simulink model "UAM_Status"  (R2024b)
settings: Solver=FixedStepAuto  StartTime=0.0  StopTime=10.0  RelTol=1e-3
libraries: simulink x1
settings Model: DataDictionary=UAM_data.sldd  Creator=admin  LastModifiedBy=admin
settings OptimizationCC: DefaultParameterBehavior=Inlined  EnhancedBackFolding=on  PassReuseOutputArgsAs=Individual arguments  ZeroExternalMemoryAtStartup=off  ZeroInternalMemoryAtStartup=off  OptimizeBlockOrder=speed  DifferentSizesBufferReuse=on  OptimizationCustomize=off  EfficientTunableParamExpr=on
settings DebuggingCC: ParameterTunabilityLossMsg=error
settings HardwareCC: ProdBitPerLong=64  ProdLargestAtomicInteger=LongLong  ProdLargestAtomicFloat=Double  ProdLongLongMode=on  ProdHWDeviceType=ARM Compatible->ARM Cortex-A (64-bit)
settings SFSimCC: MATLABDynamicMemAlloc=off
settings RTWCC: Description=Embedded Coder  SystemTargetFile=ert.tlc  TemplateMakefile=ert_default_tmf  Toolchain=Linaro AArch64 Linux v6.3.1
settings CodeAppCC: ForceParamTrailComments=on  IgnoreCustomStorageClasses=off  OperatorAnnotations=on  SimulinkDataObjDesc=on  SFDataObjDesc=on  CustomSymbolStrGlobalVar=STAT_$N$M  CustomSymbolStrType=STAT_$N$M_T  CustomSymbolStrField=STAT_$N$M  CustomSymbolStrFcn=STAT_$N$M$F  CustomSymbolStrBlkIO=STAT_rtb_$N$M  CustomSymbolStrTmpVar=STAT_tmp_$N$M  CustomSymbolStrMacro=STAT_$N$M_MACRO  InsertBlockDesc=on
settings ERTTargetCC: TargetLangStandard=C99 (ISO)  GenerateSampleERTMain=on  ERTCustomFileTemplate=example_file_process.tlc

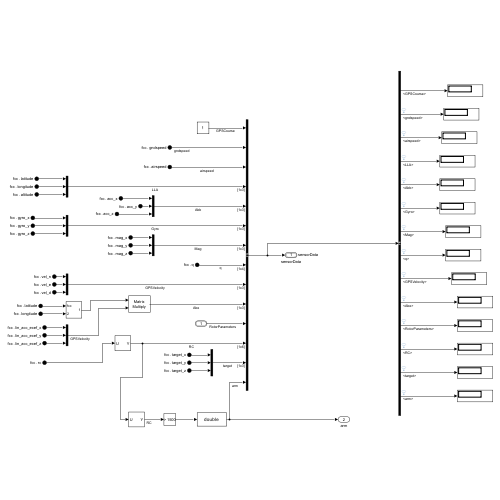
[thumbnail: Simulink's stored preview of the top-level diagram]
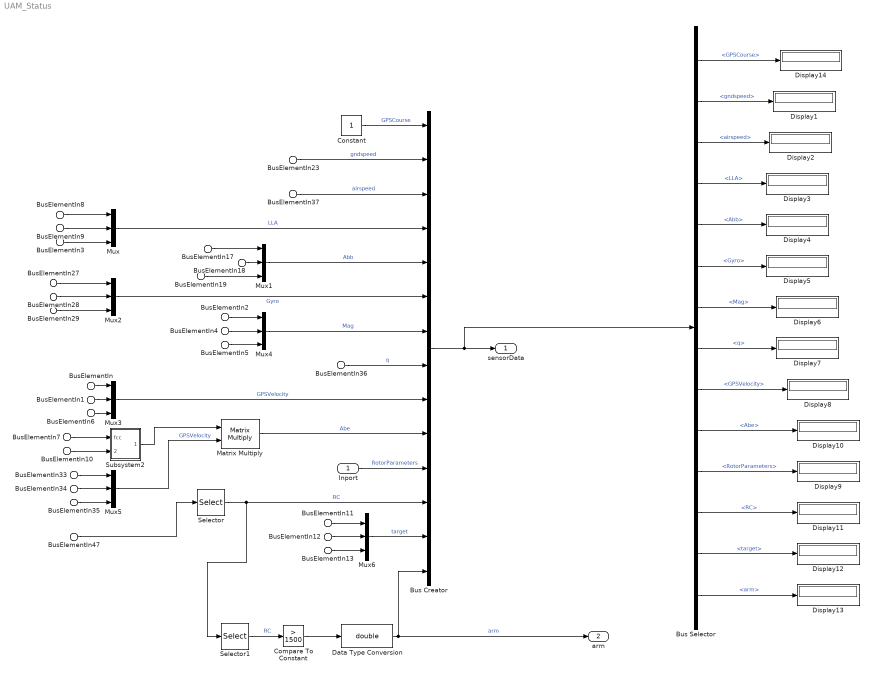
== system UAM_Status ==
  Inport : Inport  OutDataTypeStr=Bus: RotorParameters
  BusElementIn3 : Inport  Port=2  PortName=fcc  Element=altitude
  BusElementIn8 : Inport  Port=2  PortName=fcc  Element=latitude
  BusElementIn7 : Inport  Port=2  PortName=fcc  Element=latitude
  BusElementIn9 : Inport  Port=2  PortName=fcc  Element=longitude
  BusElementIn10 : Inport  Port=2  PortName=fcc  Element=longitude
  BusElementIn17 : Inport  Port=2  PortName=fcc  Element=acc_x
  BusElementIn18 : Inport  Port=2  PortName=fcc  Element=acc_y
  BusElementIn19 : Inport  Port=2  PortName=fcc  Element=acc_z
  BusElementIn : Inport  Port=2  PortName=fcc  Element=vel_n
  BusElementIn1 : Inport  Port=2  PortName=fcc  Element=vel_e
  BusElementIn6 : Inport  Port=2  PortName=fcc  Element=vel_d
  BusElementIn23 : Inport  Port=2  PortName=fcc  Element=gndspeed
  BusElementIn11 : Inport  Port=2  PortName=fcc  Element=target_x
  BusElementIn12 : Inport  Port=2  PortName=fcc  Element=target_y
  BusElementIn13 : Inport  Port=2  PortName=fcc  Element=target_z
  BusElementIn27 : Inport  Port=2  PortName=fcc  Element=gyro_x
  BusElementIn28 : Inport  Port=2  PortName=fcc  Element=gyro_y
  BusElementIn29 : Inport  Port=2  PortName=fcc  Element=gyro_z
  BusElementIn2 : Inport  Port=2  PortName=fcc  Element=mag_x
  BusElementIn4 : Inport  Port=2  PortName=fcc  Element=mag_y
  BusElementIn5 : Inport  Port=2  PortName=fcc  Element=mag_z
  BusElementIn33 : Inport  Port=2  PortName=fcc  Element=lin_acc_ecef_x
  BusElementIn34 : Inport  Port=2  PortName=fcc  Element=lin_acc_ecef_y
  BusElementIn35 : Inport  Port=2  PortName=fcc  Element=lin_acc_ecef_z
  BusElementIn36 : Inport  Port=2  PortName=fcc  Element=q
  BusElementIn37 : Inport  Port=2  PortName=fcc  Element=airspeed
  BusElementIn47 : Inport  Port=2  PortName=fcc  Element=rc
  Bus Creator : BusCreator  Inputs=14  OutDataTypeStr=Bus: sensorData
  Bus Selector : BusSelector  OutputSignals=GPSCourse,gndspeed,airspeed,LLA,Abb,Gyro,Mag,q,GPSVelocity,Abe,RotorParameters,RC,target,arm
  Compare To Constant : simulink/Logic and Bit Operations/Compare To Constant  relop=>  const=1500  OutDataTypeStr=boolean
  Constant : Constant
  Data Type Conversion : DataTypeConversion  OutDataTypeStr=double  SaturateOnIntegerOverflow=off  RndMeth=Floor
  Display{1..14} (14 alike) : Display
  Matrix Multiply : Product  Multiplication=Matrix(*)
  Mux{,1..6} (7 alike) : Mux  Inputs=3
  Selector : Selector  InputPortWidth=16  IndexOptions=Index vector (dialog)  Indices=[1:6]  OutputSizes=1
  Selector1 : Selector  InputPortWidth=6  IndexOptions=Index vector (dialog)  Indices=6  OutputSizes=1
  Subsystem2 : Subsystem
  sensorData : Outport  SignalName=sensorData  OutDataTypeStr=Bus: sensorData
  arm : Outport  Port=2
  wires:
  Selector/1 -> Bus Creator/12, Selector1/1  "RC"
  Constant/1 -> Bus Creator/1  "GPSCourse"
  BusElementIn37/1 -> Bus Creator/3  "airspeed"
  Mux/1 -> Bus Creator/4  "LLA"
  BusElementIn8/1 -> Mux/1
  BusElementIn9/1 -> Mux/2
  BusElementIn3/1 -> Mux/3
  Mux1/1 -> Bus Creator/5  "Abb"
  BusElementIn17/1 -> Mux1/1
  BusElementIn18/1 -> Mux1/2
  BusElementIn19/1 -> Mux1/3
  BusElementIn27/1 -> Mux2/1
  BusElementIn28/1 -> Mux2/2
  BusElementIn29/1 -> Mux2/3
  BusElementIn47/1 -> Selector/1
  Selector1/1 -> Compare To Constant/1  "RC"
  Compare To Constant/1 -> Data Type Conversion/1
  Data Type Conversion/1 -> Bus Creator/14, arm/1  "arm"
  Mux3/1 -> Bus Creator/9  "GPSVelocity"
  BusElementIn6/1 -> Mux3/3
  BusElementIn/1 -> Mux3/1
  BusElementIn1/1 -> Mux3/2
  BusElementIn36/1 -> Bus Creator/8  "q"
  Mux2/1 -> Bus Creator/6  "Gyro"
  Mux4/1 -> Bus Creator/7  "Mag"
  BusElementIn2/1 -> Mux4/1
  BusElementIn4/1 -> Mux4/2
  BusElementIn5/1 -> Mux4/3
  Inport/1 -> Bus Creator/11  "RotorParameters"
  BusElementIn23/1 -> Bus Creator/2  "gndspeed"
  Bus Creator/1 -> Bus Selector/1, sensorData/1
  BusElementIn33/1 -> Mux5/1
  BusElementIn34/1 -> Mux5/2
  BusElementIn35/1 -> Mux5/3
  BusElementIn7/1 -> Subsystem2/1(fcc)
  BusElementIn10/1 -> Subsystem2/2(In2)
  Subsystem2/1(Out1) -> Matrix Multiply/1
  Mux5/1 -> Matrix Multiply/2  "GPSVelocity"
  Matrix Multiply/1 -> Bus Creator/10  "Abe"
  BusElementIn11/1 -> Mux6/1
  BusElementIn12/1 -> Mux6/2
  BusElementIn13/1 -> Mux6/3
  Mux6/1 -> Bus Creator/13  "target"
  Bus Selector/1 -> Display14/1  "<GPSCourse>"
  Bus Selector/2 -> Display1/1  "<gndspeed>"
  Bus Selector/3 -> Display2/1  "<airspeed>"
  Bus Selector/4 -> Display3/1  "<LLA>"
  Bus Selector/5 -> Display4/1  "<Abb>"
  Bus Selector/6 -> Display5/1  "<Gyro>"
  Bus Selector/7 -> Display6/1  "<Mag>"
  Bus Selector/8 -> Display7/1  "<q>"
  Bus Selector/9 -> Display8/1  "<GPSVelocity>"
  Bus Selector/10 -> Display10/1  "<Abe>"
  Bus Selector/11 -> Display9/1  "<RotorParameters>"
  Bus Selector/14 -> Display13/1  "<arm>"
  Bus Selector/13 -> Display12/1  "<target>"
  Bus Selector/12 -> Display11/1  "<RC>"

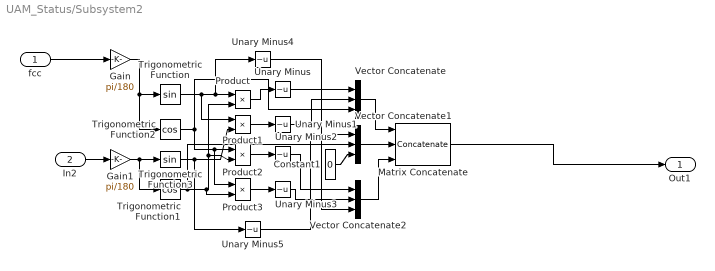
== system UAM_Status/Subsystem2 ==
  fcc : Inport
  In2 : Inport  Port=2
  Constant1 : Constant  Value=0
  Gain : Gain  Gain=pi/180
  Gain1 : Gain  Gain=pi/180
  Matrix Concatenate : Concatenate  NumInputs=3  Mode=Multidimensional array  ConcatenateDimension=2
  Product{,1..3} (4 alike) : Product
  Trigonometric Function : Trigonometry
  Trigonometric Function1 : Trigonometry  Operator=cos
  Trigonometric Function2 : Trigonometry  Operator=cos
  Trigonometric Function3 : Trigonometry
  Unary Minus{,1..5} (6 alike) : UnaryMinus
  Vector Concatenate : Concatenate  NumInputs=3
  Vector Concatenate1 : Concatenate  NumInputs=3
  Vector Concatenate2 : Concatenate  NumInputs=3
  Out1 : Outport
  wires:
  Product3/1 -> Unary Minus3/1
  Vector Concatenate/1 -> Matrix Concatenate/1
  Trigonometric Function1/1 -> Vector Concatenate1/2, Product3/2, Product/2, Product2/2
  Unary Minus4/1 -> Vector Concatenate2/3
  Vector Concatenate2/1 -> Matrix Concatenate/3
  Trigonometric Function3/1 -> Unary Minus5/1, Product1/2
  Trigonometric Function/1 -> Product1/1, Unary Minus4/1, Product/1
  Gain/1 -> Trigonometric Function2/1, Trigonometric Function/1
  Product/1 -> Unary Minus/1
  Vector Concatenate1/1 -> Matrix Concatenate/2
  Trigonometric Function2/1 -> Product2/1, Product3/1, Vector Concatenate/3
  fcc/1 -> Gain/1
  Gain1/1 -> Trigonometric Function1/1, Trigonometric Function3/1
  Constant1/1 -> Vector Concatenate1/3
  Unary Minus5/1 -> Vector Concatenate1/1
  In2/1 -> Gain1/1
  Unary Minus2/1 -> Vector Concatenate2/1
  Product2/1 -> Unary Minus2/1
  Product1/1 -> Unary Minus1/1
  Unary Minus/1 -> Vector Concatenate/1
  Unary Minus1/1 -> Vector Concatenate/2
  Unary Minus3/1 -> Vector Concatenate2/2
  Matrix Concatenate/1 -> Out1/1
